simulink model "PP_241015_1_PT1_PH"  (R2016b)
settings: Solver=FixedStepAuto  StartTime=0.0  StopTime=0.4  RelTol=1e-3
undefined symbols (not defined in the file): DiscIntNeverNeededParam
libraries: powerlib x20, simulink x2, simulink_extras x2
settings Model: Creator=Anton  LastModifiedBy=Victor

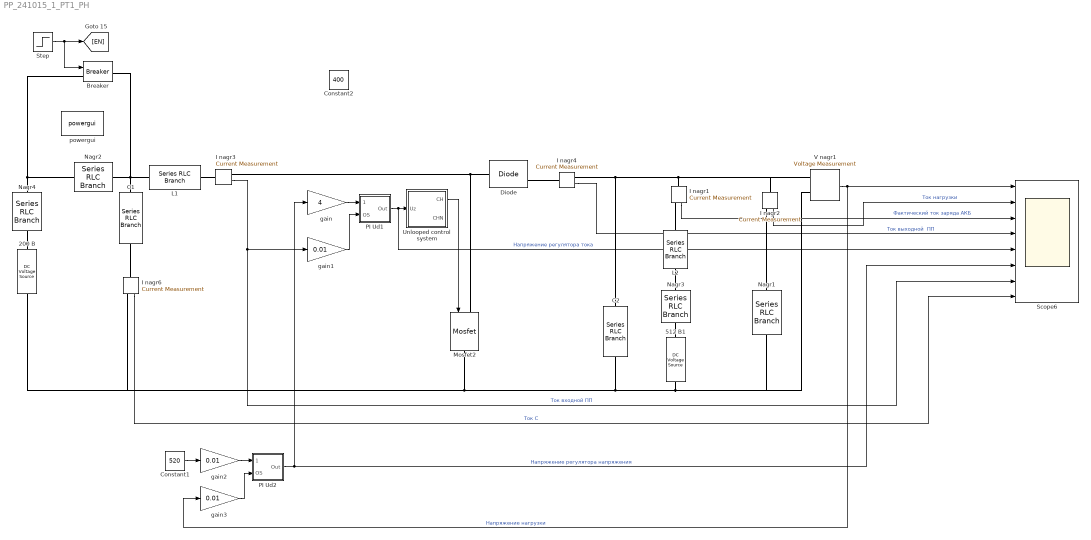
== system PP_241015_1_PT1_PH ==
  200 В : powerlib/Electrical Sources/DC Voltage Source  Amplitude=200  Measurements=None
  512 В1 : powerlib/Electrical Sources/DC Voltage Source  Amplitude=512  Measurements=None
  Breaker : powerlib/Elements/Breaker  InitialState=0  SwitchingTimes="[1/60  5/60]"  External=on  BreakerResistance=0.0001  SnubberResistance=1e6  SnubberCapacitance=inf  Measurements=None  MoreParameters=on  NoBreakLoop=off
  C1 : powerlib/Elements/Series RLC Branch  LConnTagsString=__new0  RConnTagsString=__new0  BranchType=C  Resistance=1e-6  Inductance=1e-3  SetiL0=off  InitialCurrent=0  Capacitance=4e-3  Setx0=on  InitialVoltage=200  Measurements=Branch voltage
  C2 : powerlib/Elements/Series RLC Branch  LConnTagsString=__new0  RConnTagsString=__new0  BranchType=C  Resistance=1e-6  Inductance=1e-3  SetiL0=off  InitialCurrent=0  Capacitance=8e-3  Setx0=on  InitialVoltage=200  Measurements=Branch voltage
  Constant1 : Constant  Value=520
  Constant2 : Constant  Value=400
  Diode : powerlib/Power Electronics/Diode  Ron=0.001  Lon=0  Vf=0.8  IC=0  UseSnubber=off  Rs=500  Cs=250e-9  Measurements=on
  I nagr{1..4,6} (5 alike) : powerlib/Measurements/Current Measurement  PhasorSimulation=off  OutputType=Complex  PSBequivalent=0
  L1 : powerlib/Elements/Series RLC Branch  LConnTagsString=__new0  RConnTagsString=__new0  BranchType=L  Resistance=0.001  Inductance=5e-4  SetiL0=off  InitialCurrent=0  Capacitance=1e-6  Setx0=off  InitialVoltage=0  Measurements=None
  L2 : powerlib/Elements/Series RLC Branch  LConnTagsString=__new0  RConnTagsString=__new0  BranchType=L  Resistance=0.001  Inductance=1e-3  SetiL0=off  InitialCurrent=0  Capacitance=1e-6  Setx0=off  InitialVoltage=0  Measurements=None
  Mosfet2 : powerlib/Power Electronics/Mosfet  Ron=1e-6  Lon=0  Rd=1e-6  Vfd=0  IC=0  Rs=1e5  Cs=inf  Measurements=off
  Nagr1 : powerlib/Elements/Series RLC Branch  LConnTagsString=__new0  RConnTagsString=__new0  BranchType=R  Resistance=400  Inductance=1e-3  SetiL0=off  InitialCurrent=0  Capacitance=1e-6  Setx0=off  InitialVoltage=0  Measurements=None
  Nagr2 : powerlib/Elements/Series RLC Branch  LConnTagsString=__new0  RConnTagsString=__new0  BranchType=R  Resistance=5  Inductance=1e-3  SetiL0=off  InitialCurrent=0  Capacitance=1e-6  Setx0=off  InitialVoltage=0  Measurements=None
  Nagr3 : powerlib/Elements/Series RLC Branch  LConnTagsString=__new0  RConnTagsString=__new0  BranchType=R  Resistance=0.05  Inductance=1e-3  SetiL0=off  InitialCurrent=0  Capacitance=1e-6  Setx0=off  InitialVoltage=0  Measurements=None
  Nagr4 : powerlib/Elements/Series RLC Branch  LConnTagsString=__new0  RConnTagsString=__new0  BranchType=R  Resistance=0.05  Inductance=1e-3  SetiL0=off  InitialCurrent=0  Capacitance=1e-6  Setx0=off  InitialVoltage=0  Measurements=None
  PI Ud1 : Subsystem
  PI Ud2 : Subsystem
  Scope6 : Scope  NumInputPorts=8
  Step : Step  Time=0.0  SampleTime=0
  Unlooped control system : Subsystem
  V nagr1 : powerlib/Measurements/Voltage Measurement  PhasorSimulation=off  OutputType=Complex  PSBequivalent=0
  gain : Gain  Gain=4  SaturateOnIntegerOverflow=on  OutDataTypeStr=Inherit: Same as input  ParamDataTypeStr=Inherit: Same as input
  gain1 : Gain  Gain=0.01  SaturateOnIntegerOverflow=on  OutDataTypeStr=Inherit: Same as input  ParamDataTypeStr=Inherit: Same as input
  gain2 : Gain  Gain=0.01  SaturateOnIntegerOverflow=on  OutDataTypeStr=Inherit: Same as input  ParamDataTypeStr=Inherit: Same as input
  gain3 : Gain  Gain=0.01  SaturateOnIntegerOverflow=on  OutDataTypeStr=Inherit: Same as input  ParamDataTypeStr=Inherit: Same as input
  powergui : powerlib/powergui  Priority=1  SimulationMode=Discrete  SolverType=Tustin/Backward Euler (TBE)  SampleTime=1e-6  frequency=60  SPID=off  DisableSnubberDevices=off  DisableRonSwitches=off  DisableVfSwitches=off  SwTol=0  DisplayEquations=off  Interpol=off  ExternalGateDelay=off  methode=off  Ts=10  FunctionMessages=off  echomessages=off  HookPort=off  EnableUseOfTLC=off  x0status=blocks  frequencyindice=0  Pbase=100e6  ErrMax=1e-4  Iterations=50  UnitsV=kV  UnitsW=MW  buscounter=0  RestoreLinks=warning  ResistiveCurrentMeasurement=off  Frange=[0:2:500]  Ylog=off  Xlog=on  ShowGrid=off  save=off  variable=ZData  structure=0  ZoomFFT=off  StartTime=0.0  cycles=1  DisplayStyle=1  fundamental=60  FreqAxis=off  MaxFrequency=1000  frequencyindicesteady=1  RmsSteady=1  display=off
  wires:
  V nagr1/1 -> Scope6/1, gain3/1  "Напряжение нагрузки"
  Step/1 -> Breaker/1, [EN]
  I nagr3/1 -> gain1/1, Scope6/7  "Ток входной ПП"
  I nagr6/1 -> Scope6/8  "Ток С"
  I nagr2/1 -> Scope6/2  "Ток нагрузки"
  I nagr1/1 -> Scope6/3  "Фактический ток заряда АКБ"
  I nagr4/1 -> Scope6/4  "Ток выходной  ПП"
  gain/1 -> PI Ud1/1(Zad)
  gain1/1 -> PI Ud1/2(OS)
  Unlooped control system/1(CH) -> Mosfet2/1
  gain2/1 -> PI Ud2/1(Zad)
  gain3/1 -> PI Ud2/2(OS)
  Constant1/1 -> gain2/1
  PI Ud2/1(Out) -> gain/1, Scope6/6  "Напряжение регулятора напряжения"
  PI Ud1/1(Out) -> Scope6/5, Unlooped control system/1(Uz)  "Напряжение регулятора тока"
  connections:
  V nagr1/LConn2 -- Nagr1/RConn1 -- 512 В1/LConn1 -- C2/RConn1 -- I nagr6/RConn1 -- 200 В/LConn1 -- Mosfet2/RConn1
  Diode/LConn1 -- I nagr3/RConn1 -- Mosfet2/LConn1
  L1/RConn1 -- I nagr3/LConn1
  C2/LConn1 -- V nagr1/LConn1 -- I nagr2/LConn1 -- I nagr1/LConn1 -- I nagr4/RConn1
  Breaker/LConn1 -- Nagr4/LConn1 -- Nagr2/RConn1
  I nagr6/LConn1 -- C1/RConn1
  I nagr4/LConn1 -- Diode/RConn1
  Nagr4/RConn1 -- 200 В/RConn1
  I nagr2/RConn1 -- Nagr1/LConn1
  Nagr2/LConn1 -- C1/LConn1 -- Breaker/RConn1 -- L1/LConn1
  512 В1/RConn1 -- Nagr3/RConn1
  L2/LConn1 -- Nagr3/LConn1
  L2/RConn1 -- I nagr1/RConn1

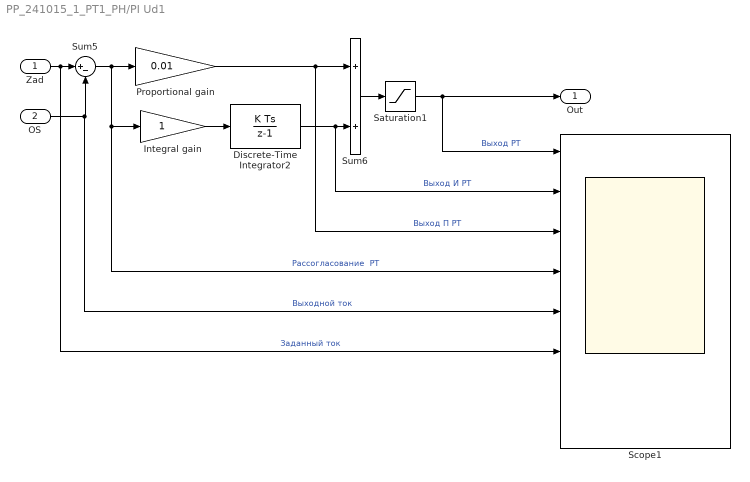
== system PP_241015_1_PT1_PH/PI Ud1 ==
  Zad : Inport
  OS : Inport  Port=2
  Discrete-Time Integrator2 : DiscreteIntegrator  SampleTime=-1  LimitOutput=on  UpperSaturationLimit=1  LowerSaturationLimit=0  ICPrevOutput=DiscIntNeverNeededParam  ICPrevScaledInput=DiscIntNeverNeededParam
  Integral gain : Gain  SaturateOnIntegerOverflow=on  OutDataTypeStr=Inherit: Same as input  ParamDataTypeStr=Inherit: Same as input
  Proportional gain : Gain  Gain=0.01  SaturateOnIntegerOverflow=on  OutDataTypeStr=Inherit: Same as input  ParamDataTypeStr=Inherit: Same as input
  Saturation1 : Saturate  UpperLimit=0.97  LowerLimit=0.05
  Scope1 : Scope  NumInputPorts=8
  Sum5 : Sum  Inputs=|+-  SaturateOnIntegerOverflow=on  InputSameDT=on  OutDataTypeStr=Inherit: Same as first input
  Sum6 : Sum  SaturateOnIntegerOverflow=on  InputSameDT=on  OutDataTypeStr=Inherit: Same as first input
  Out : Outport
  wires:
  Integral gain/1 -> Discrete-Time Integrator2/1
  Proportional gain/1 -> Scope1/3, Sum6/1  "Выход П РТ"
  Discrete-Time Integrator2/1 -> Scope1/2, Sum6/2  "Выход И РТ"
  OS/1 -> Scope1/5, Sum5/2  "Выходной ток"
  Zad/1 -> Scope1/6, Sum5/1  "Заданный ток"
  Sum5/1 -> Scope1/4, Integral gain/1, Proportional gain/1  "Рассогласование  РТ"
  Sum6/1 -> Saturation1/1
  Saturation1/1 -> Out/1, Scope1/1  "Выход РТ"

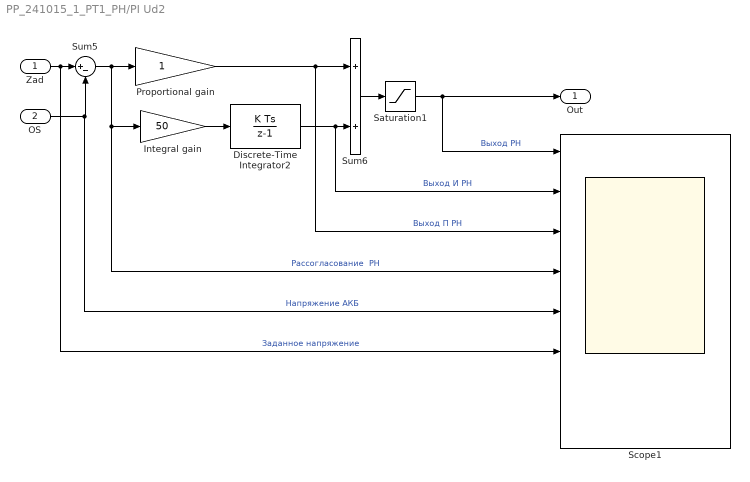
== system PP_241015_1_PT1_PH/PI Ud2 ==
  Zad : Inport
  OS : Inport  Port=2
  Discrete-Time Integrator2 : DiscreteIntegrator  SampleTime=-1  LimitOutput=on  UpperSaturationLimit=1  LowerSaturationLimit=0  ICPrevOutput=DiscIntNeverNeededParam  ICPrevScaledInput=DiscIntNeverNeededParam
  Integral gain : Gain  Gain=50  SaturateOnIntegerOverflow=on  OutDataTypeStr=Inherit: Same as input  ParamDataTypeStr=Inherit: Same as input
  Proportional gain : Gain  SaturateOnIntegerOverflow=on  OutDataTypeStr=Inherit: Same as input  ParamDataTypeStr=Inherit: Same as input
  Saturation1 : Saturate  UpperLimit=0.97  LowerLimit=0.03
  Scope1 : Scope  NumInputPorts=8
  Sum5 : Sum  Inputs=|+-  SaturateOnIntegerOverflow=on  InputSameDT=on  OutDataTypeStr=Inherit: Same as first input
  Sum6 : Sum  SaturateOnIntegerOverflow=on  InputSameDT=on  OutDataTypeStr=Inherit: Same as first input
  Out : Outport
  wires:
  Integral gain/1 -> Discrete-Time Integrator2/1
  Proportional gain/1 -> Scope1/3, Sum6/1  "Выход П РН"
  Discrete-Time Integrator2/1 -> Scope1/2, Sum6/2  "Выход И РН"
  OS/1 -> Scope1/5, Sum5/2  "Напряжение АКБ"
  Zad/1 -> Scope1/6, Sum5/1  "Заданное напряжение"
  Sum5/1 -> Scope1/4, Integral gain/1, Proportional gain/1  "Рассогласование  РН"
  Sum6/1 -> Saturation1/1
  Saturation1/1 -> Out/1, Scope1/1  "Выход РН"

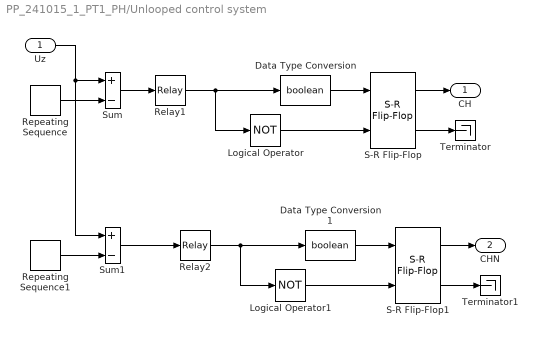
== system PP_241015_1_PT1_PH/Unlooped control system ==
  Uz : Inport
  Data Type Conversion : DataTypeConversion  OutDataTypeStr=boolean
  Data Type Conversion1 : DataTypeConversion  OutDataTypeStr=boolean
  Logical Operator : Logic  Operator=NOT  AllPortsSameDT=off  OutDataTypeStr=boolean
  Logical Operator1 : Logic  Operator=NOT  AllPortsSameDT=off  OutDataTypeStr=boolean
  Relay1 : Relay  OnSwitchValue=0.01  OffSwitchValue=-0.01
  Relay2 : Relay  OnSwitchValue=0.01  OffSwitchValue=-0.01
  Repeating Sequence : simulink/Sources/Repeating Sequence  rep_seq_t="[0  0.0000625 0.000125]"  rep_seq_y=[0 1 0]
  Repeating Sequence1 : simulink/Sources/Repeating Sequence  rep_seq_t="[0  0.0000625 0.000125]"  rep_seq_y=[1 0 1]
  S-R Flip-Flop : simulink_extras/Flip Flops/S-R Flip-Flop  initial_condition=0
  S-R Flip-Flop1 : simulink_extras/Flip Flops/S-R Flip-Flop  initial_condition=0
  Sum : Sum  Inputs=+-
  Sum1 : Sum  Inputs=+-
  Terminator : Terminator
  Terminator1 : Terminator
  CH : Outport
  CHN : Outport  Port=2
  wires:
  S-R Flip-Flop/1 -> CH/1
  Data Type Conversion/1 -> S-R Flip-Flop/1
  Logical Operator/1 -> S-R Flip-Flop/2
  Relay1/1 -> Logical Operator/1, Data Type Conversion/1
  Repeating Sequence/1 -> Sum/2
  Uz/1 -> Sum1/1, Sum/1
  Sum/1 -> Relay1/1
  S-R Flip-Flop/2 -> Terminator/1
  Repeating Sequence1/1 -> Sum1/2
  S-R Flip-Flop1/1 -> CHN/1
  Data Type Conversion1/1 -> S-R Flip-Flop1/1
  Logical Operator1/1 -> S-R Flip-Flop1/2
  Relay2/1 -> Logical Operator1/1, Data Type Conversion1/1
  S-R Flip-Flop1/2 -> Terminator1/1
  Sum1/1 -> Relay2/1
